simulink model "plantasimulacao"  (R2023a)
settings: Solver=VariableStepAuto  StartTime=0.0  StopTime=20  RelTol=1e-3
settings Model: Creator=Mateus  LastModifiedBy=Mateus

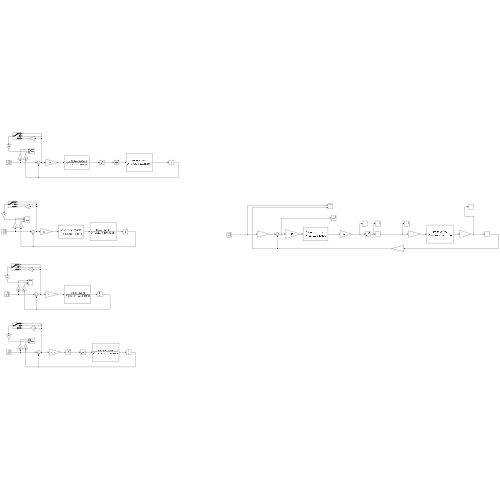
[thumbnail: Simulink's stored preview of the top-level diagram]
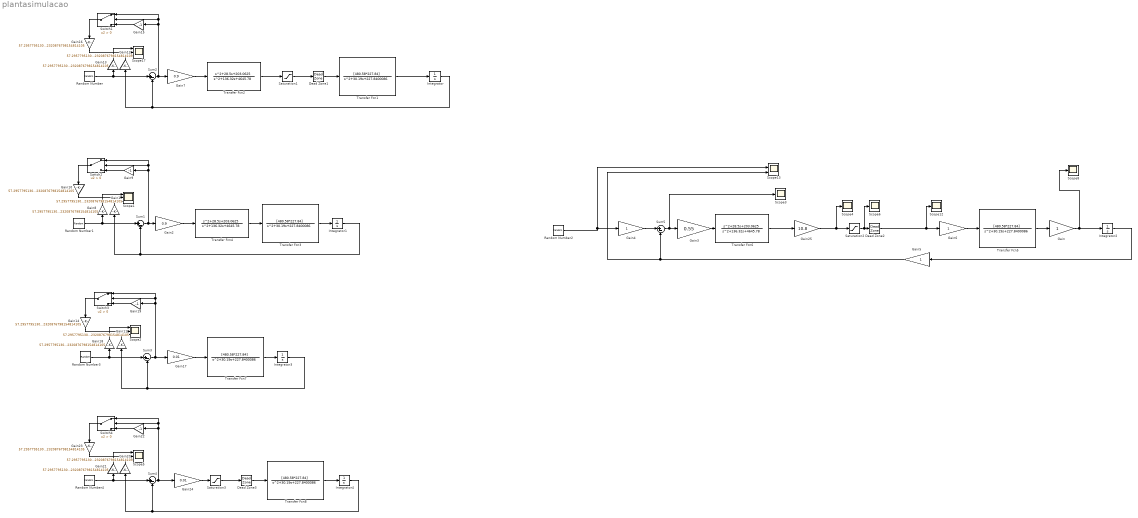
== system plantasimulacao ==
  Dead Zone1 : DeadZone  LowerValue=-40/255  UpperValue=40/255
  Dead Zone2 : DeadZone  LowerValue=0  UpperValue=40/255
  Dead Zone3 : DeadZone  LowerValue=-40/255  UpperValue=40/255
  Gain{,4..6} (4 alike) : Gain
  Gain{1,8,10..14,16,18,20..21,23} (12 alike) : Gain  Gain=57.295779513082320876798154814105
  Gain{9,15,19,22} (4 alike) : Gain  Gain=-1
  Gain17 : Gain  Gain=0.01
  Gain2 : Gain  Gain=0.9
  Gain24 : Gain  Gain=0.01
  Gain25 : Gain  Gain=10.8
  Gain3 : Gain  Gain=0.55
  Gain7 : Gain  Gain=0.9
  Integrator{,1..4} (5 alike) : Integrator
  Random Number{,1..4} (5 alike) : RandomNumber  Variance=6.28  Seed=7  SampleTime=2
  Saturation1 : Saturate  UpperLimit=1  LowerLimit=-1  OutMin=[-1]  OutMax=[1]
  Saturation2 : Saturate  UpperLimit=1  LowerLimit=-1  OutMin=[-1]  OutMax=[1]
  Saturation3 : Saturate  UpperLimit=1  LowerLimit=-1  OutMin=[-1]  OutMax=[1]
  Scope{1..2,5,17} (4 alike) : Scope  NumInputPorts=3
  Scope{3..4,6,8,12} (5 alike) : Scope
  Scope13 : Scope  NumInputPorts=2
  Sum{1..5} (5 alike) : Sum  Inputs=|+-
  Switch{1..4} (4 alike) : Switch  Criteria=u2 > Threshold  SaturateOnIntegerOverflow=off  InputSameDT=off
  Transfer Fcn{1,3,5,7..8} (5 alike) : TransferFcn  Numerator=[480.58*227.84]  Denominator=[1 30.19 227.8400086]
  Transfer Fcn2 : TransferFcn  Numerator=[1 28.5 203.0625]  Denominator=[1 136.32 4645.78]
  Transfer Fcn4 : TransferFcn  Numerator=[1 28.5 203.0625]  Denominator=[1 136.32 4645.78]
  Transfer Fcn6 : TransferFcn  Numerator=[1 28.5 203.0625]  Denominator=[1 136.32 4645.78]
  wires:
  Saturation1/1 -> Dead Zone1/1
  Sum2/1 -> Gain7/1, Gain15/1, Switch1/1, Switch1/2
  Gain7/1 -> Transfer Fcn2/1
  Integrator/1 -> Sum2/2, Gain12/1
  Random Number/1 -> Gain13/1, Sum2/1
  Integrator1/1 -> Gain1/1, Sum1/2
  Random Number1/1 -> Gain8/1, Sum1/1
  Gain2/1 -> Transfer Fcn4/1
  Integrator2/1 -> Gain5/1
  Random Number2/1 -> Scope13/1, Gain4/1
  Dead Zone2/1 -> Gain6/1, Scope12/1
  Saturation2/1 -> Scope6/1, Dead Zone2/1
  Gain3/1 -> Transfer Fcn6/1
  Sum5/1 -> Scope3/1, Gain3/1
  Transfer Fcn6/1 -> Gain25/1
  Transfer Fcn5/1 -> Gain/1
  Gain4/1 -> Sum5/1
  Gain5/1 -> Scope13/2, Sum5/2
  Gain6/1 -> Transfer Fcn5/1
  Gain/1 -> Integrator2/1, Scope8/1
  Transfer Fcn3/1 -> Integrator1/1
  Transfer Fcn1/1 -> Integrator/1
  Transfer Fcn2/1 -> Saturation1/1
  Transfer Fcn4/1 -> Transfer Fcn3/1
  Gain12/1 -> Scope17/3
  Gain13/1 -> Scope17/1
  Gain15/1 -> Switch1/3
  Switch1/1 -> Gain16/1
  Gain16/1 -> Scope17/2
  Dead Zone1/1 -> Transfer Fcn1/1
  Switch2/1 -> Gain10/1
  Sum1/1 -> Gain9/1, Switch2/1, Switch2/2, Gain2/1
  Gain1/1 -> Scope1/3
  Gain8/1 -> Scope1/1
  Gain9/1 -> Switch2/3
  Gain10/1 -> Scope1/2
  Gain17/1 -> Transfer Fcn7/1
  Switch3/1 -> Gain14/1
  Gain11/1 -> Scope2/3
  Gain18/1 -> Scope2/1
  Transfer Fcn7/1 -> Integrator3/1
  Gain14/1 -> Scope2/2
  Integrator3/1 -> Gain11/1, Sum3/2
  Gain19/1 -> Switch3/3
  Random Number3/1 -> Gain18/1, Sum3/1
  Sum3/1 -> Gain19/1, Switch3/1, Switch3/2, Gain17/1
  Dead Zone3/1 -> Transfer Fcn8/1
  Switch4/1 -> Gain23/1
  Gain20/1 -> Scope5/3
  Gain21/1 -> Scope5/1
  Gain24/1 -> Saturation3/1
  Gain22/1 -> Switch4/3
  Gain23/1 -> Scope5/2
  Random Number4/1 -> Gain21/1, Sum4/1
  Sum4/1 -> Gain24/1, Gain22/1, Switch4/1, Switch4/2
  Integrator4/1 -> Sum4/2, Gain20/1
  Transfer Fcn8/1 -> Integrator4/1
  Saturation3/1 -> Dead Zone3/1
  Gain25/1 -> Scope4/1, Saturation2/1
